simulink model "Cruise_Control_Model"  (R2020a)
settings: Solver=ode45  StartTime=0.0  StopTime=120  RelTol=1e-3
undefined symbols (not defined in the file): b, m, Ts
settings Model: DataDictionary=CruiseCtrl_data.sldd  Creator=NIKITA  LastModifiedBy=NIKITA
settings DebuggingCC: ModelReferenceExtraNoncontSigs=none

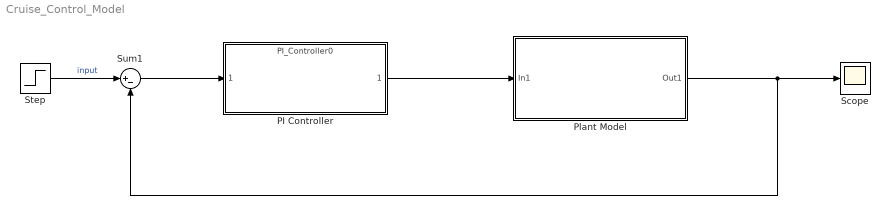
== system Cruise_Control_Model ==
  PI Controller : ModelReference  ModelNameDialog=PI_Controller0  ModelReferenceVersion=1.17
  Plant Model : Subsystem
  "Scope " : Scope
  "Step " : Step  Time=0  After=u  SampleTime=Ts
  Sum1 : Sum  Inputs=|+-
  wires:
  Plant Model/1("Out1 ") -> "Scope "/1, Sum1/2
  "Step "/1 -> Sum1/1  "input"
  Sum1/1 -> PI Controller/1
  PI Controller/1 -> Plant Model/1("In1 ")

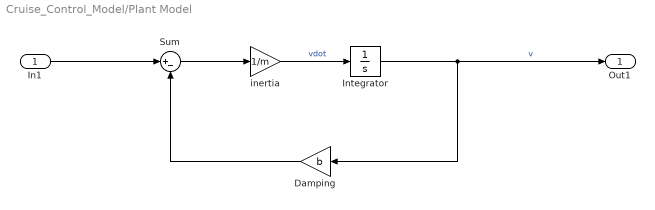
== system Cruise_Control_Model/Plant Model ==
  "In1 " : Inport
  Damping : Gain  Gain=b
  "Integrator " : Integrator
  Sum : Sum  Inputs=|+-
  inertia : Gain  Gain=1/m
  "Out1 " : Outport
  wires:
  Sum/1 -> inertia/1
  "In1 "/1 -> Sum/1
  inertia/1 -> "Integrator "/1  "vdot"
  "Integrator "/1 -> "Out1 "/1, Damping/1  "v"
  Damping/1 -> Sum/2
